simulink model "controller_simulation"  (R2022b)
settings: Solver=VariableStepAuto  StartTime=0.0  StopTime=10  RelTol=1e-3
values from neighbouring files (symbols this model uses):
  b = 2    [controller_simulation_.m]
  Ip = 1.5    [controller_simulation_.m]
  Ir = 1    [controller_simulation_.m]
  Kd = 1    [controller_simulation_.m]
  Ki = 5    [controller_simulation_.m]
  Kp = 5    [controller_simulation_.m]
libraries: slpidlib x1
settings Model: Creator=krzy5z70f  LastModifiedBy=krzy5z70f

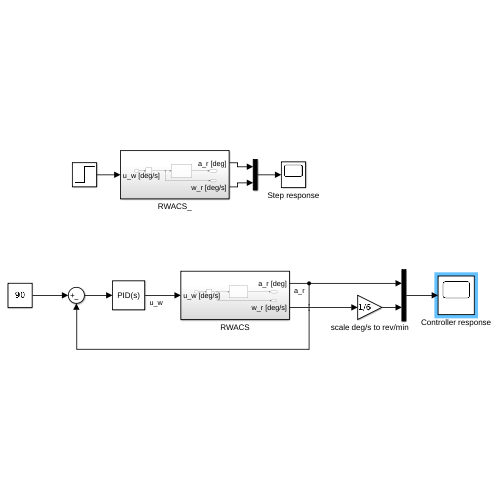
[thumbnail: Simulink's stored preview of the top-level diagram]
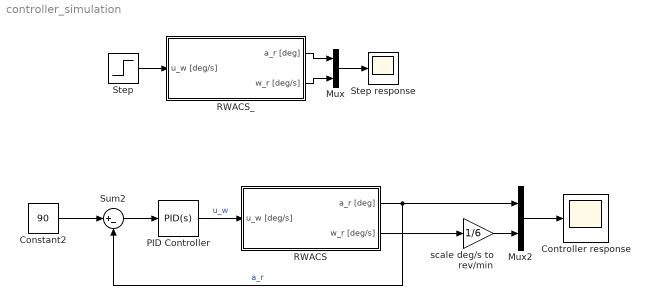
== system controller_simulation ==
  Constant2 : Constant  Value=90
  Controller response : Scope
  Mux : Mux  Inputs=2
  Mux2 : Mux  Inputs=2
  PID Controller : slpidlib/PID Controller  Controller=PID  Form=Parallel  TimeDomain=Continuous-time  UseExternalTs=off  SampleTime=-1  IntegratorMethod=Forward Euler  FilterMethod=Forward Euler  ControllerParametersSource=internal  P=Kp  I=Ki  UseKiTs=off  D=Kd  N=100  UseFilter=on  TunerSelectOption=Transfer Function Based (PID Tuner App)  InitialConditionSource=internal  InitialConditionForIntegrator=0  InitialConditionForFilter=0  DifferentiatorICPrevScaledInput=0  ExternalReset=none  TrackingMode=off  Kt=1  LimitOutput=off  SatLimitsSource=internal  UpperSaturationLimit=inf  LowerSaturationLimit=-inf  LinearizeAsGain=on  AntiWindupMode=none  Kb=1  LimitIntegrator=off  UpperIntegratorSaturationLimit=inf  LowerIntegratorSaturationLimit=-inf  POutMin=[]  POutMax=[]  IOutMin=[]  IOutMax=[]  DOutMin=[]  DOutMax=[]  NOutMin=[]  NOutMax=[]  SumOutMin=[]  SumOutMax=[]  SaturationOutMin=[]  SaturationOutMax=[]  PParamMin=[]  PParamMax=[]  IParamMin=[]  IParamMax=[]  DParamMin=[]  DParamMax=[]  NParamMin=[]  NParamMax=[]  KbParamMin=[]  KbParamMax=[]  KtParamMin=[]  KtParamMax=[]  KbOutMin=[]  KbOutMax=[]  KtOutMin=[]  KtOutMax=[]  IntegratorOutMin=[]  IntegratorOutMax=[]  FilterOutMin=[]  FilterOutMax=[]  SumI1OutMin=[]  SumI1OutMax=[]  SumI2OutMin=[]  SumI2OutMax=[]  SumI3OutMin=[]  SumI3OutMax=[]  SumI4OutMin=[]  SumI4OutMax=[]  SumDOutMin=[]  SumDOutMax=[]  DifferentiatorOutMin=[]  DifferentiatorOutMax=[]  FilterDiffOutCoefMin=[]  FilterDiffOutCoefMax=[]  ReciprocalOutMin=[]  ReciprocalOutMax=[]  SumDenOutMin=[]  SumDenOutMax=[]  SumNumOutMin=[]  SumNumOutMax=[]  DivideOutMin=[]  DivideOutMax=[]  UdiffTsProdOutMin=[]  UdiffTsProdOutMax=[]  NTsProdOutMin=[]  NTsProdOutMax=[]  UintegralTsProdOutMin=[]  UintegralTsProdOutMax=[]  UngainTsProdOutMin=[]  UngainTsProdOutMax=[]  ClampingZeroOutDataTypeStr=Inherit: Inherit via back propagation  ClampingZeroOutMin=[]  ClampingZeroOutMax=[]  FilterDenConstantOutDataTypeStr=Inherit: Inherit via back propagation  FilterDenConstantOutMin=[]  FilterDenConstantOutMax=[]  PCopyOutDataTypeStr=Inherit: Inherit via back propagation  PCopyOutMin=[]  PCopyOutMax=[]  NCopyOutDataTypeStr=Inherit: Inherit via back propagation  NCopyOutMin=[]  NCopyOutMax=[]  IntegratorContinuousStateAttributes=''  IntegratorStateMustResolveToSignalObject=off  IntegratorRTWStateStorageClass=Auto  FilterContinuousStateAttributes=''  FilterStateMustResolveToSignalObject=off  FilterRTWStateStorageClass=Auto  ParallelPVariant=InternalParameters  IdealPVariant=Disabled  IVariant=InternalParameters  DVariant=InternalParameters  IntegratorVariant=Continuous  SatVariant=Disabled  AWVariant=Passthrough  PCopyVariant=Disabled  TRVariant=Disabled  FdbkBlocksVariant=Forward  IdealPFdbkVariant=Disabled  SatFdbkVariant=Disabled  DerivativeFilterVariant=ContFilter  NVariant=InternalParameters  NCopyVariant=Disabled  FilterICVariant=InternalICsFilter  IntegratorICVariant=InternalICs  ExternalResetVariant=Disabled  TRSumVariant=Passthrough  SumFdbkVariant=Disabled  SumVariant=Sum_PID  TsampFilterVariant=InternalTs  TsampNgainVariant=Passthrough  TsampIntegralVariant=Passthrough  ExternalSaturationOutDataTypeStr=Inherit: Same as second input
  RWACS : Subsystem
  RWACS_ : Subsystem
  Step : Step  After=1200  SampleTime=0
  Step response : Scope
  Sum2 : Sum  Inputs=|+-
  scale deg/s to rev/min : Gain  Gain=1/6
  wires:
  Step/1 -> RWACS_/1(u_w [deg/s])
  Mux/1 -> Step response/1
  RWACS_/2(w_r [deg/s]) -> Mux/2
  RWACS_/1(a_r [deg]) -> Mux/1
  Constant2/1 -> Sum2/1
  Sum2/1 -> PID Controller/1
  PID Controller/1 -> RWACS/1(u_w [deg/s])  "u_w"
  RWACS/1(a_r [deg]) -> Mux2/1, Sum2/2  "a_r"
  Mux2/1 -> Controller response/1
  RWACS/2(w_r [deg/s]) -> scale deg/s to rev/min/1
  scale deg/s to rev/min/1 -> Mux2/2

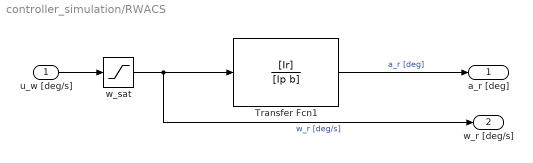
== system controller_simulation/RWACS ==
  u_w [deg/s] : Inport
  Transfer Fcn1 : TransferFcn  Numerator=[Ir]  Denominator=[Ip b]
  w_sat : Saturate  UpperLimit=2400  LowerLimit=-2400
  a_r [deg] : Outport
  w_r [deg/s] : Outport  Port=2
  wires:
  w_sat/1 -> Transfer Fcn1/1, w_r [deg/s]/1  "w_r [deg/s]"
  Transfer Fcn1/1 -> a_r [deg]/1  "a_r [deg]"
  u_w [deg/s]/1 -> w_sat/1

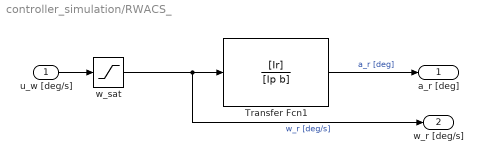
== system controller_simulation/RWACS_ ==
  u_w [deg/s] : Inport
  Transfer Fcn1 : TransferFcn  Numerator=[Ir]  Denominator=[Ip b]
  w_sat : Saturate  UpperLimit=2400  LowerLimit=-2400
  a_r [deg] : Outport
  w_r [deg/s] : Outport  Port=2
  wires:
  Transfer Fcn1/1 -> a_r [deg]/1  "a_r [deg]"
  u_w [deg/s]/1 -> w_sat/1
  w_sat/1 -> w_r [deg/s]/1, Transfer Fcn1/1  "w_r [deg/s]"
